simulink model "StraightWithLeadingCar_cs"  (R2016a)
settings: Solver=ode5  SolverMode=SingleTasking  StartTime=0.0  StopTime=40  FixedStep=1/1000  RelTol=1e-3
PreLoadFcn:
  | mbxruntime.callbacks.PreLoadFcn(bdroot);
PostLoadFcn:
  | mbxruntime.callbacks.PostLoadFcn(bdroot);
InitFcn:
  | mbxruntime.callbacks.InitFcn(bdroot);
StartFcn:
  | mbxruntime.callbacks.StartFcn(bdroot);
StopFcn:
  | mbxruntime.callbacks.StopFcn(bdroot);
model workspace (MAT data in the model file):
  mbox_table : struct (value not decoded)
  model_closed = 0
  sim_status = 0
values from neighbouring files (symbols this model uses):
  ACCDuration = 5    [PreScan_Runscript.m]
  V0 = ACCArray(2*ACCCasei-1)    [PreScan_Runscript.m]
  V1 = ACCArray(2*ACCCasei)    [PreScan_Runscript.m]
  VAccuracyIn = 0.8    [PreScan_Runscript.m]
  VDurationIn = 2    [PreScan_Runscript.m]
  VPIDIn = ACCArray(2*ACCCasei-1)    [PreScan_Runscript.m]
  VToleranceIn = 1    [PreScan_Runscript.m]
undefined symbols (not defined in the file or in its folder): ADASID, BMotor1, BMotor2, BrkDelayTime, DControlB, Delay1, Delay2, DiscIntNeverNeededParam, IControlB, JMotor1, JMotor2, mbxruntime, PControlB, PreScanCarSimLoadFcn, ratioGearF, ratioGearR, tabledata, TorqDelayTime, Tstep
undefined symbols (not defined in the file): SteeringColumn, SteeringWheel, WheelL0, WheelL1, WheelR0, WheelR1
libraries: simulink x14, simulink_extras x11, PreScanSimulinkLibrary x9, MyLib x3, Solver_SF x2, PreScanUsefulBlocks x2, pil_lib x1
(part 10 of 12)

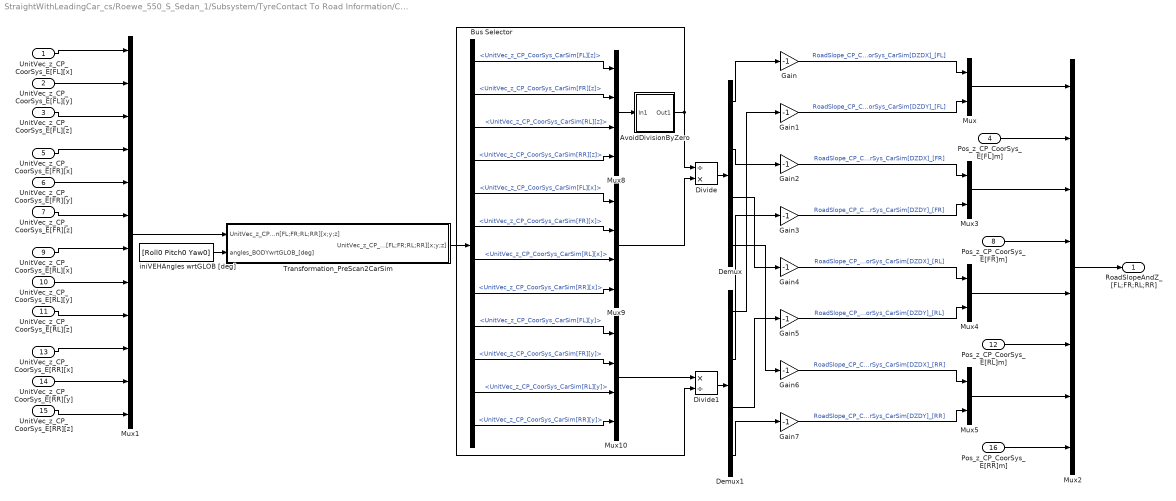
== system StraightWithLeadingCar_cs/Roewe_550_S_Sedan_1/Subsystem/TyreContact To Road Information/Contact To Road Information ==
  UnitVec_z_CP_CoorSys_E[FL][x] : Inport
  UnitVec_z_CP_CoorSys_E[FL][y] : Inport  Port=2
  UnitVec_z_CP_CoorSys_E[FL][z] : Inport  Port=3
  " Pos_z_CP_CoorSys_E[FL]m]" : Inport  Port=4
  UnitVec_z_CP_CoorSys_E[FR][x] : Inport  Port=5
  UnitVec_z_CP_CoorSys_E[FR][y] : Inport  Port=6
  UnitVec_z_CP_CoorSys_E[FR][z] : Inport  Port=7
  " Pos_z_CP_CoorSys_E[FR]m]" : Inport  Port=8
  UnitVec_z_CP_CoorSys_E[RL][x] : Inport  Port=9
  UnitVec_z_CP_CoorSys_E[RL][y] : Inport  Port=10
  UnitVec_z_CP_CoorSys_E[RL][z] : Inport  Port=11
  " Pos_z_CP_CoorSys_E[RL]m]" : Inport  Port=12
  UnitVec_z_CP_CoorSys_E[RR][x] : Inport  Port=13
  UnitVec_z_CP_CoorSys_E[RR][y] : Inport  Port=14
  UnitVec_z_CP_CoorSys_E[RR][z] : Inport  Port=15
  " Pos_z_CP_CoorSys_E[RR]m]" : Inport  Port=16
  AvoidDivisionByZero : Subsystem
  Bus Selector : BusSelector  OutputSignals=UnitVec_z_CP_CoorSys_CarSim[FL][x;y;z].UnitVec_z_CP_CoorSys_CarSim[FL][z],UnitVec_z_CP_CoorSys_CarSim[FR][x;y;z].UnitVec_z_CP_CoorSys_CarSim[FR][z],UnitVec_z_CP_CoorSys_CarSim[RL][x;y;z].UnitVec_z_CP_CoorSys_CarSim[RL][z],UnitVec_z_CP_CoorSys_CarSim[RR][x;y;z].UnitVec_z_CP_CoorSys_CarSim[RR][z],UnitVec_z_CP_CoorSys_CarSim[FL][x;y;z].UnitVec_z_CP_CoorSys_CarSim[FL][x],UnitVec_z_CP_CoorSys_CarSim[FR][x;y;z].UnitVec_z_CP_CoorSys_CarSim[FR][x],UnitVec_z_CP_CoorSys_CarSim[RL][x;y;z].UnitVec_z_CP_CoorSys_CarSim[RL][x],UnitVec_z_CP_CoorSys_CarSim[RR][x;y;z].UnitVec_z_CP_CoorSys_CarSim[RR][x],UnitVec_z_CP_CoorSys_CarSim[FL][x;y;z].UnitVec_z_CP_CoorSys_CarSim[FL][y],UnitVec_z_CP_CoorSys_CarSim[FR][x;y;z].UnitVec_z_CP_CoorSys_CarSim[FR][y],UnitVec_z_CP_CoorSys_CarSim[RL][x;y;z].UnitVec_z_CP_CoorSys_CarSim[RL][y],UnitVec_z_CP_CoorSys_CarSim[RR][x;y;z].UnitVec_z_CP_CoorSys_CarSim[RR][y]
  Demux : Demux
  Demux1 : Demux
  Divide : Product  Inputs=/*
  Divide1 : Product  Inputs=*/
  Gain{,1..7} (8 alike) : Gain  Gain=-1
  Mux{,3..5} (4 alike) : Mux  Inputs=2
  Mux1 : Mux  Inputs=12
  Mux10 : Mux
  Mux2 : Mux  Inputs=[2 1 2 1 2 1 2 1]
  Mux8 : Mux
  Mux9 : Mux
  Transformation_PreScan2CarSim : Subsystem
  iniVEHAngles wrtGLOB [deg] : Constant  Value=[Roll0 Pitch0 Yaw0]
  RoadSlopeAndZ_[FL;FR;RL;RR] : Outport
  wires:
  AvoidDivisionByZero/1(Out1) -> Divide1/2, Divide/1
  Demux1/4 -> Gain7/1
  Demux/4 -> Gain6/1
  Demux1/3 -> Gain5/1
  Demux/3 -> Gain4/1
  Demux1/2 -> Gain3/1
  Demux/2 -> Gain2/1
  Demux/1 -> Gain/1
  Demux1/1 -> Gain1/1
  Divide1/1 -> Demux1/1
  Divide/1 -> Demux/1
  Mux10/1 -> Divide1/1
  Mux9/1 -> Divide/2
  Mux8/1 -> AvoidDivisionByZero/1(In1)
  Bus Selector/12 -> Mux10/4  "<UnitVec_z_CP_CoorSys_CarSim[RR][y]>"
  Bus Selector/11 -> Mux10/3  "<UnitVec_z_CP_CoorSys_CarSim[RL][y]>"
  Bus Selector/10 -> Mux10/2  "<UnitVec_z_CP_CoorSys_CarSim[FR][y]>"
  Bus Selector/9 -> Mux10/1  "<UnitVec_z_CP_CoorSys_CarSim[FL][y]>"
  Bus Selector/8 -> Mux9/4  "<UnitVec_z_CP_CoorSys_CarSim[RR][x]>"
  Bus Selector/7 -> Mux9/3  "<UnitVec_z_CP_CoorSys_CarSim[RL][x]>"
  Bus Selector/6 -> Mux9/2  "<UnitVec_z_CP_CoorSys_CarSim[FR][x]>"
  Bus Selector/5 -> Mux9/1  "<UnitVec_z_CP_CoorSys_CarSim[FL][x]>"
  Bus Selector/4 -> Mux8/4  "<UnitVec_z_CP_CoorSys_CarSim[RR][z]>"
  Bus Selector/3 -> Mux8/3  "<UnitVec_z_CP_CoorSys_CarSim[RL][z]>"
  Bus Selector/2 -> Mux8/2  "<UnitVec_z_CP_CoorSys_CarSim[FR][z]>"
  Bus Selector/1 -> Mux8/1  "<UnitVec_z_CP_CoorSys_CarSim[FL][z]>"
  Mux5/1 -> Mux2/7
  Mux4/1 -> Mux2/5
  Mux3/1 -> Mux2/3
  " Pos_z_CP_CoorSys_E[FL]m]"/1 -> Mux2/2
  Mux/1 -> Mux2/1
  Gain/1 -> Mux/1  "RoadSlope_CP_CoorSys_CarSim[DZDX]_[FL]"
  " Pos_z_CP_CoorSys_E[RR]m]"/1 -> Mux2/8
  " Pos_z_CP_CoorSys_E[RL]m]"/1 -> Mux2/6
  " Pos_z_CP_CoorSys_E[FR]m]"/1 -> Mux2/4
  Transformation_PreScan2CarSim/1(UnitVec_z_CP_CoorSys _CarSim[FL;FR;RL;RR][x;y;z]) -> Bus Selector/1
  UnitVec_z_CP_CoorSys_E[RR][z]/1 -> Mux1/12
  UnitVec_z_CP_CoorSys_E[RR][y]/1 -> Mux1/11
  UnitVec_z_CP_CoorSys_E[RR][x]/1 -> Mux1/10
  UnitVec_z_CP_CoorSys_E[RL][z]/1 -> Mux1/9
  UnitVec_z_CP_CoorSys_E[RL][y]/1 -> Mux1/8
  UnitVec_z_CP_CoorSys_E[RL][x]/1 -> Mux1/7
  UnitVec_z_CP_CoorSys_E[FR][z]/1 -> Mux1/6
  UnitVec_z_CP_CoorSys_E[FR][y]/1 -> Mux1/5
  UnitVec_z_CP_CoorSys_E[FR][x]/1 -> Mux1/4
  UnitVec_z_CP_CoorSys_E[FL][z]/1 -> Mux1/3
  UnitVec_z_CP_CoorSys_E[FL][y]/1 -> Mux1/2
  UnitVec_z_CP_CoorSys_E[FL][x]/1 -> Mux1/1
  Mux1/1 -> Transformation_PreScan2CarSim/1(UnitVec_z_CP_CoorSys_PreScan[FL;FR;RL;RR][x;y;z])
  iniVEHAngles wrtGLOB [deg]/1 -> Transformation_PreScan2CarSim/2(angles_BODYwrtGLOB_[deg])
  Mux2/1 -> RoadSlopeAndZ_[FL;FR;RL;RR]/1
  Gain1/1 -> Mux/2  "RoadSlope_CP_CoorSys_CarSim[DZDY]_[FL]"
  Gain2/1 -> Mux3/1  "RoadSlope_CP_CoorSys_CarSim[DZDX]_[FR]"
  Gain3/1 -> Mux3/2  "RoadSlope_CP_CoorSys_CarSim[DZDY]_[FR]"
  Gain4/1 -> Mux4/1  "RoadSlope_CP_CoorSys_CarSim[DZDX]_[RL]"
  Gain5/1 -> Mux4/2  "RoadSlope_CP_CoorSys_CarSim[DZDY]_[RL]"
  Gain6/1 -> Mux5/1  "RoadSlope_CP_CoorSys_CarSim[DZDX]_[RR]"
  Gain7/1 -> Mux5/2  "RoadSlope_CP_CoorSys_CarSim[DZDY]_[RR]"

== system StraightWithLeadingCar_cs/Roewe_550_S_Sedan_1/Subsystem1/CarSim2PreScanSTATE/Transformation_SprungMassCarSim2PreScan ==
  In1 : Inport
  Demux : Demux  Outputs=3
  Ini z-position VEHICLE wrt GLOBAL axis system [m] : Constant  Value=z0
  Mux : Mux  Inputs=3
  Sum1 : Sum  Inputs=+-
  Out1 : Outport
  wires:
  Mux/1 -> Out1/1
  Ini z-position VEHICLE wrt GLOBAL axis system [m]/1 -> Sum1/2
  Demux/1 -> Mux/1
  Sum1/1 -> Mux/3
  Demux/3 -> Sum1/1
  Demux/2 -> Mux/2
  In1/1 -> Demux/1

== system StraightWithLeadingCar_cs/Roewe_550_S_Sedan_1/Subsystem1/CarSim2PreScan_BUS/Steering ==
  SteeringWheel_In : Inport
  AvoidDivisionByZero : Subsystem
  Bus Creator4 : BusCreator  Inputs=1
  DefaultValue : Constant  Value=16
  Demux2 : Demux  Outputs=2
  Divide : Product  Inputs=*/
  Switch : Switch  Criteria=u2 ~= 0
  Steering : Outport
  wires:
  AvoidDivisionByZero/1(Out1) -> Divide/2
  Switch/1 -> Bus Creator4/1  "SteeringRatio_[-]"
  DefaultValue/1 -> Switch/3
  Divide/1 -> Switch/1, Switch/2  "Steering_Ration[-]"
  Demux2/2 -> AvoidDivisionByZero/1(In1)  "Axle1ReducedSW"
  Demux2/1 -> Divide/1  "SteeringWheelAngle_[deg]"
  Bus Creator4/1 -> Steering/1  "Steering"
  SteeringWheel_In/1 -> Demux2/1

== system StraightWithLeadingCar_cs/Roewe_550_S_Sedan_1/Subsystem1/CarSim2PreScan_BUS/Vehicle ==
  v_VehicleCoG[x;y;z][km|h] : Inport
  Bus Creator1 : BusCreator  Inputs=1
  Bus Creator7 : BusCreator  Inputs=1
  Bus Creator8 : BusCreator  Inputs=3
  Demux : Demux  Outputs=3
  Vehicle : Outport
  wires:
  Demux/3 -> Bus Creator8/3  "v_Vehicle[z][km|h]"
  Demux/2 -> Bus Creator8/2  "v_Vehicle[y][km|h]"
  Demux/1 -> Bus Creator8/1  "v_Vehicle[x][km|h]"
  Bus Creator7/1 -> Bus Creator1/1  "Velocities"
  Bus Creator8/1 -> Bus Creator7/1  "Linear"
  Bus Creator1/1 -> Vehicle/1  "Vehicle"
  v_VehicleCoG[x;y;z][km|h]/1 -> Demux/1

== system StraightWithLeadingCar_cs/Roewe_550_S_Sedan_1/Subsystem1/CarSim2PreScan_BUS/Wheel ==
  SprungMass_Pos_Global[x;y;z][m] : Inport
  SprungMass_Angle_Global[x;y;z][deg] : Inport  Port=2
  CarSim_Pos_Wheel_[FL;FR;RL;RR][x;y;z][m] : Inport  Port=3
  CarSim_Angle_Wheel_[FL;FR;RL;RR][x;y;z][deg;rev;deg] : Inport  Port=4
  Bus Creator3 : BusCreator  Inputs=2
  Bus Creator6 : BusCreator  Inputs=1
  Convert CarSim to PreScan Wheel Position : Subsystem
  Convert CarSim to PreScan Wheel Rotation : Subsystem
  Demux : Demux  Outputs=[3 3 3 3]
  Demux1 : Demux  Outputs=[3 3 3 3]
  Wheel : Outport
  wires:
  SprungMass_Angle_Global[x;y;z][deg]/1 -> Convert CarSim to PreScan Wheel Rotation/5(Angle_Vehicle[x;y;z][deg]), Convert CarSim to PreScan Wheel Position/2(SprungMass_Angle_Global[x;y;z][deg])
  SprungMass_Pos_Global[x;y;z][m]/1 -> Convert CarSim to PreScan Wheel Position/1(SprungMass_Pos_Global[x;y;z][m])
  CarSim_Angle_Wheel_[FL;FR;RL;RR][x;y;z][deg;rev;deg]/1 -> Demux1/1
  Demux1/4 -> Convert CarSim to PreScan Wheel Rotation/4(CarSim_Angle_RR_Wheel_CoorSys_V[deg;rev;deg])  "CarSim_Angle_RR_Wheel_CoorSys_V[deg;rev;deg]"
  Demux1/3 -> Convert CarSim to PreScan Wheel Rotation/3(CarSim_Angle_RL_Wheel_CoorSys_V[deg;rev;deg])  "CarSim_Angle_RL_Wheel_CoorSys_V[deg;rev;deg]"
  Demux1/2 -> Convert CarSim to PreScan Wheel Rotation/2(CarSim_Angle_FR_Wheel_CoorSys_V[deg;rev;deg])  "CarSim_Angle_FR_Wheel_CoorSys_V[deg;rev;deg]"
  Demux1/1 -> Convert CarSim to PreScan Wheel Rotation/1(CarSim_Angle_FL_Wheel_CoorSys_V[deg;rev;deg])  "CarSim_Angle_FL_Wheel_CoorSys_V[deg;rev;deg]"
  CarSim_Pos_Wheel_[FL;FR;RL;RR][x;y;z][m]/1 -> Demux/1
  Demux/4 -> Convert CarSim to PreScan Wheel Position/6(CarSim_Pos_RR_Wheel[x;y;z][m])  "CarSim_Pos_RR_Wheel[x;y;z][m]"
  Demux/3 -> Convert CarSim to PreScan Wheel Position/5(CarSim_Pos_RL_Wheel[x;y;z][m])  "CarSim_Pos_RL_Wheel[x;y;z][m]"
  Demux/2 -> Convert CarSim to PreScan Wheel Position/4(CarSim_Pos_FR_Wheel[x;y;z][m])  "CarSim_Pos_FR_Wheel[x;y;z][m]"
  Demux/1 -> Convert CarSim to PreScan Wheel Position/3(CarSim_Pos_FL_Wheel[x;y;z][m])  "CarSim_Pos_FL_Wheel[x;y;z][m]"
  Bus Creator6/1 -> Wheel/1  "Wheel"
  Bus Creator3/1 -> Bus Creator6/1  "Position"
  Convert CarSim to PreScan Wheel Rotation/1(PreScanWheel_Rot) -> Bus Creator3/2
  Convert CarSim to PreScan Wheel Position/1(PreScanWheel_Pos) -> Bus Creator3/1

== system StraightWithLeadingCar_cs/BMW_X5_SUV_1/Trajectories/Traj2State1/Traj2State2/MuxState ==
  x [m] : Inport
  y [m] : Inport  Port=2
  z [m] : Inport  Port=3
  dx [m/s] : Inport  Port=4
  dy [m/s] : Inport  Port=5
  dz [m/s] : Inport  Port=6
  R [rad] : Inport  Port=7
  P [rad] : Inport  Port=8
  Y [rad] : Inport  Port=9
  Mux : Mux  Inputs=9
  state : Outport
  wires:
  z [m]/1 -> Mux/3
  y [m]/1 -> Mux/2
  x [m]/1 -> Mux/1
  Y [rad]/1 -> Mux/9
  P [rad]/1 -> Mux/8
  R [rad]/1 -> Mux/7
  dz [m/s]/1 -> Mux/6
  dy [m/s]/1 -> Mux/5
  dx [m/s]/1 -> Mux/4
  Mux/1 -> state/1

== system StraightWithLeadingCar_cs/BMW_X5_SUV_1/Trajectories/Traj2State1/Traj2State2/Traj2MuxState_Ext ==
  Traj : Inport
  Terminator{1..9} (9 alike) : Terminator
  demux : Subsystem
  x [m] : Outport
  y [m] : Outport  Port=2
  z [m] : Outport  Port=3
  dx [m/s] : Outport  Port=4
  dy [m/s] : Outport  Port=5
  dz [m/s] : Outport  Port=6
  R [rad] : Outport  Port=7
  P [rad] : Outport  Port=8
  Y [rad] : Outport  Port=9
  wires:
  demux/9(Y) -> Y [rad]/1
  demux/7(R) -> R [rad]/1
  demux/5(vely) -> dy [m/s]/1
  demux/4(velx) -> dx [m/s]/1
  demux/10(velR) -> Terminator4/1
  demux/11(velP) -> Terminator5/1
  demux/12(velY) -> Terminator1/1
  demux/13(accx) -> Terminator8/1
  demux/14(accy) -> Terminator9/1
  demux/15(accz) -> Terminator7/1
  demux/18(accY) -> Terminator2/1
  demux/16(accR) -> Terminator3/1
  demux/17(accP) -> Terminator6/1
  demux/3(z) -> z [m]/1
  Traj/1 -> demux/1(traj)
  demux/6(velz) -> dz [m/s]/1
  demux/1(x) -> x [m]/1
  demux/2(y) -> y [m]/1
  demux/8(P) -> P [rad]/1

== system StraightWithLeadingCar_cs/Roewe_550_S_Sedan_1/CarSim I//O/PreScanLaneMarker/Subsystem/Sensor Data ==
  Sensor Data : Inport
  Bus Selector : BusSelector  OutputSignals=ScanAtSensor.LeftLaneIntersection2.WorldCoordinateY,ScanAtDistance1.LeftLaneIntersection2.WorldCoordinateY,ScanAtDistance2.LeftLaneIntersection2.WorldCoordinateY,ScanAtDistance3.LeftLaneIntersection2.WorldCoordinateY
  Bus Selector1 : BusSelector  OutputSignals=ScanAtSensor.LeftLaneIntersection1.WorldCoordinateY,ScanAtDistance1.LeftLaneIntersection1.WorldCoordinateY,ScanAtDistance2.LeftLaneIntersection1.WorldCoordinateY,ScanAtDistance3.LeftLaneIntersection1.WorldCoordinateY
  Bus Selector2 : BusSelector  OutputSignals=ScanAtSensor.RightLaneIntersection1.WorldCoordinateY,ScanAtDistance1.RightLaneIntersection1.WorldCoordinateY,ScanAtDistance2.RightLaneIntersection1.WorldCoordinateY,ScanAtDistance3.RightLaneIntersection1.WorldCoordinateY
  Bus Selector3 : BusSelector  OutputSignals=ScanAtSensor.RightLaneIntersection2.WorldCoordinateX,ScanAtDistance1.RightLaneIntersection2.WorldCoordinateX,ScanAtDistance2.RightLaneIntersection2.WorldCoordinateX,ScanAtDistance3.RightLaneIntersection2.WorldCoordinateX
  Bus Selector4 : BusSelector  OutputSignals=ScanAtSensor.SliceCenterCoordsX,ScanAtSensor.SliceCenterCoordsY
  Bus Selector5 : BusSelector  OutputSignals=ScanAtSensor.LeftLaneIntersection2.WorldCoordinateX,ScanAtDistance1.LeftLaneIntersection2.WorldCoordinateX,ScanAtDistance2.LeftLaneIntersection2.WorldCoordinateX,ScanAtDistance3.LeftLaneIntersection2.WorldCoordinateX
  Bus Selector6 : BusSelector  OutputSignals=ScanAtSensor.LeftLaneIntersection1.WorldCoordinateX,ScanAtDistance1.LeftLaneIntersection1.WorldCoordinateX,ScanAtDistance2.LeftLaneIntersection1.WorldCoordinateX,ScanAtDistance3.LeftLaneIntersection1.WorldCoordinateX
  Bus Selector7 : BusSelector  OutputSignals=ScanAtSensor.RightLaneIntersection1.WorldCoordinateX,ScanAtDistance1.RightLaneIntersection1.WorldCoordinateX,ScanAtDistance2.RightLaneIntersection1.WorldCoordinateX,ScanAtDistance3.RightLaneIntersection1.WorldCoordinateX
  Bus Selector8 : BusSelector  OutputSignals=ScanAtSensor.RightLaneIntersection2.WorldCoordinateY,ScanAtDistance1.RightLaneIntersection2.WorldCoordinateY,ScanAtDistance2.RightLaneIntersection2.WorldCoordinateY,ScanAtDistance3.RightLaneIntersection2.WorldCoordinateY
  Mux{,1..7} (8 alike) : Mux
  X0 : Outport
  Y0 : Outport  Port=2
  Lane3_X_Part0 : Outport  Port=3
  Lane1_X_Part0 : Outport  Port=4
  Lane2_X_Part0 : Outport  Port=5
  Lane4_X_Part0 : Outport  Port=6
  Lane3_Y_Part0 : Outport  Port=7
  Lane1_Y_Part0 : Outport  Port=8
  Lane2_Y_Part0 : Outport  Port=9
  Lane4_Y_Part0 : Outport  Port=10
  wires:
  Sensor Data/1 -> Bus Selector8/1, Bus Selector2/1, Bus Selector1/1, Bus Selector/1, Bus Selector3/1, Bus Selector5/1, Bus Selector4/1, Bus Selector6/1, Bus Selector7/1
  Bus Selector4/2 -> Y0/1  "<SliceCenterCoordsY>"
  Bus Selector4/1 -> X0/1  "<SliceCenterCoordsX>"
  Bus Selector5/2 -> Mux/2  "<WorldCoordinateX>"
  Bus Selector5/4 -> Mux/4  "<WorldCoordinateX>"
  Bus Selector5/1 -> Mux/1  "<WorldCoordinateX>"
  Bus Selector5/3 -> Mux/3  "<WorldCoordinateX>"
  Bus Selector/3 -> Mux4/3  "<WorldCoordinateY>"
  Bus Selector/4 -> Mux4/4  "<WorldCoordinateY>"
  Bus Selector/1 -> Mux4/1  "<WorldCoordinateY>"
  Bus Selector/2 -> Mux4/2  "<WorldCoordinateY>"
  Mux/1 -> Lane3_X_Part0/1
  Mux4/1 -> Lane3_Y_Part0/1
  Bus Selector6/4 -> Mux5/4  "<WorldCoordinateX>"
  Bus Selector6/3 -> Mux5/3  "<WorldCoordinateX>"
  Bus Selector6/2 -> Mux5/2  "<WorldCoordinateX>"
  Bus Selector6/1 -> Mux5/1  "<WorldCoordinateX>"
  Bus Selector1/3 -> Mux1/3  "<WorldCoordinateY>"
  Bus Selector1/2 -> Mux1/2  "<WorldCoordinateY>"
  Bus Selector1/4 -> Mux1/4  "<WorldCoordinateY>"
  Bus Selector1/1 -> Mux1/1  "<WorldCoordinateY>"
  Mux1/1 -> Lane1_Y_Part0/1
  Mux5/1 -> Lane1_X_Part0/1
  Bus Selector7/2 -> Mux2/2  "<WorldCoordinateX>"
  Bus Selector7/3 -> Mux2/3  "<WorldCoordinateX>"
  Bus Selector7/1 -> Mux2/1  "<WorldCoordinateX>"
  Bus Selector7/4 -> Mux2/4  "<WorldCoordinateX>"
  Bus Selector2/2 -> Mux3/2  "<WorldCoordinateY>"
  Bus Selector2/1 -> Mux3/1  "<WorldCoordinateY>"
  Bus Selector2/3 -> Mux3/3  "<WorldCoordinateY>"
  Bus Selector2/4 -> Mux3/4  "<WorldCoordinateY>"
  Bus Selector3/2 -> Mux6/2  "<WorldCoordinateX>"
  Bus Selector3/1 -> Mux6/1  "<WorldCoordinateX>"
  Bus Selector3/3 -> Mux6/3  "<WorldCoordinateX>"
  Bus Selector3/4 -> Mux6/4  "<WorldCoordinateX>"
  Bus Selector8/1 -> Mux7/1  "<WorldCoordinateY>"
  Bus Selector8/2 -> Mux7/2  "<WorldCoordinateY>"
  Bus Selector8/3 -> Mux7/3  "<WorldCoordinateY>"
  Bus Selector8/4 -> Mux7/4  "<WorldCoordinateY>"
  Mux3/1 -> Lane2_Y_Part0/1
  Mux7/1 -> Lane4_Y_Part0/1
  Mux2/1 -> Lane2_X_Part0/1
  Mux6/1 -> Lane4_X_Part0/1

== system StraightWithLeadingCar_cs/Roewe_550_S_Sedan_1/CarSim I//O/PreScanLaneMarker/Subsystem/Sensor Data1 ==
  Sensor Data : Inport
  Bus Selector : BusSelector  OutputSignals=ScanAtSensor.LeftLaneIntersection2.WorldCoordinateY,ScanAtDistance1.LeftLaneIntersection2.WorldCoordinateY,ScanAtDistance2.LeftLaneIntersection2.WorldCoordinateY,ScanAtDistance3.LeftLaneIntersection2.WorldCoordinateY
  Bus Selector1 : BusSelector  OutputSignals=ScanAtSensor.LeftLaneIntersection1.WorldCoordinateY,ScanAtDistance1.LeftLaneIntersection1.WorldCoordinateY,ScanAtDistance2.LeftLaneIntersection1.WorldCoordinateY,ScanAtDistance3.LeftLaneIntersection1.WorldCoordinateY
  Bus Selector2 : BusSelector  OutputSignals=ScanAtSensor.RightLaneIntersection1.WorldCoordinateY,ScanAtDistance1.RightLaneIntersection1.WorldCoordinateY,ScanAtDistance2.RightLaneIntersection1.WorldCoordinateY,ScanAtDistance3.RightLaneIntersection1.WorldCoordinateY
  Bus Selector3 : BusSelector  OutputSignals=ScanAtSensor.RightLaneIntersection2.WorldCoordinateX,ScanAtDistance1.RightLaneIntersection2.WorldCoordinateX,ScanAtDistance2.RightLaneIntersection2.WorldCoordinateX,ScanAtDistance3.RightLaneIntersection2.WorldCoordinateX
  Bus Selector5 : BusSelector  OutputSignals=ScanAtSensor.LeftLaneIntersection2.WorldCoordinateX,ScanAtDistance1.LeftLaneIntersection2.WorldCoordinateX,ScanAtDistance2.LeftLaneIntersection2.WorldCoordinateX,ScanAtDistance3.LeftLaneIntersection2.WorldCoordinateX
  Bus Selector6 : BusSelector  OutputSignals=ScanAtSensor.LeftLaneIntersection1.WorldCoordinateX,ScanAtDistance1.LeftLaneIntersection1.WorldCoordinateX,ScanAtDistance2.LeftLaneIntersection1.WorldCoordinateX,ScanAtDistance3.LeftLaneIntersection1.WorldCoordinateX
  Bus Selector7 : BusSelector  OutputSignals=ScanAtSensor.RightLaneIntersection1.WorldCoordinateX,ScanAtDistance1.RightLaneIntersection1.WorldCoordinateX,ScanAtDistance2.RightLaneIntersection1.WorldCoordinateX,ScanAtDistance3.RightLaneIntersection1.WorldCoordinateX
  Bus Selector8 : BusSelector  OutputSignals=ScanAtSensor.RightLaneIntersection2.WorldCoordinateY,ScanAtDistance1.RightLaneIntersection2.WorldCoordinateY,ScanAtDistance2.RightLaneIntersection2.WorldCoordinateY,ScanAtDistance3.RightLaneIntersection2.WorldCoordinateY
  Mux{,1..7} (8 alike) : Mux
  Lane3_X_Part1 : Outport
  Lane1_X_Part1 : Outport  Port=2
  Lane2_X_Part1 : Outport  Port=3
  Lane4_X_Part1 : Outport  Port=4
  Lane3_Y_Part1 : Outport  Port=5
  Lane1_Y_Part1 : Outport  Port=6
  Lane2_Y_Part1 : Outport  Port=7
  Lane4_Y_Part1 : Outport  Port=8
  wires:
  Sensor Data/1 -> Bus Selector8/1, Bus Selector2/1, Bus Selector1/1, Bus Selector/1, Bus Selector3/1, Bus Selector5/1, Bus Selector6/1, Bus Selector7/1
  Bus Selector5/2 -> Mux/2  "<WorldCoordinateX>"
  Bus Selector5/4 -> Mux/4  "<WorldCoordinateX>"
  Bus Selector5/1 -> Mux/1  "<WorldCoordinateX>"
  Bus Selector5/3 -> Mux/3  "<WorldCoordinateX>"
  Bus Selector/3 -> Mux4/3  "<WorldCoordinateY>"
  Bus Selector/4 -> Mux4/4  "<WorldCoordinateY>"
  Bus Selector/1 -> Mux4/1  "<WorldCoordinateY>"
  Bus Selector/2 -> Mux4/2  "<WorldCoordinateY>"
  Mux/1 -> Lane3_X_Part1/1
  Mux4/1 -> Lane3_Y_Part1/1
  Bus Selector6/4 -> Mux5/4  "<WorldCoordinateX>"
  Bus Selector6/3 -> Mux5/3  "<WorldCoordinateX>"
  Bus Selector6/2 -> Mux5/2  "<WorldCoordinateX>"
  Bus Selector6/1 -> Mux5/1  "<WorldCoordinateX>"
  Bus Selector1/3 -> Mux1/3  "<WorldCoordinateY>"
  Bus Selector1/2 -> Mux1/2  "<WorldCoordinateY>"
  Bus Selector1/4 -> Mux1/4  "<WorldCoordinateY>"
  Bus Selector1/1 -> Mux1/1  "<WorldCoordinateY>"
  Mux1/1 -> Lane1_Y_Part1/1
  Mux5/1 -> Lane1_X_Part1/1
  Bus Selector7/2 -> Mux2/2  "<WorldCoordinateX>"
  Bus Selector7/3 -> Mux2/3  "<WorldCoordinateX>"
  Bus Selector7/1 -> Mux2/1  "<WorldCoordinateX>"
  Bus Selector7/4 -> Mux2/4  "<WorldCoordinateX>"
  Bus Selector2/2 -> Mux3/2  "<WorldCoordinateY>"
  Bus Selector2/1 -> Mux3/1  "<WorldCoordinateY>"
  Bus Selector2/3 -> Mux3/3  "<WorldCoordinateY>"
  Bus Selector2/4 -> Mux3/4  "<WorldCoordinateY>"
  Bus Selector3/2 -> Mux6/2  "<WorldCoordinateX>"
  Bus Selector3/1 -> Mux6/1  "<WorldCoordinateX>"
  Bus Selector3/3 -> Mux6/3  "<WorldCoordinateX>"
  Bus Selector3/4 -> Mux6/4  "<WorldCoordinateX>"
  Bus Selector8/1 -> Mux7/1  "<WorldCoordinateY>"
  Bus Selector8/2 -> Mux7/2  "<WorldCoordinateY>"
  Bus Selector8/3 -> Mux7/3  "<WorldCoordinateY>"
  Bus Selector8/4 -> Mux7/4  "<WorldCoordinateY>"
  Mux3/1 -> Lane2_Y_Part1/1
  Mux7/1 -> Lane4_Y_Part1/1
  Mux2/1 -> Lane2_X_Part1/1
  Mux6/1 -> Lane4_X_Part1/1

== system StraightWithLeadingCar_cs/Roewe_550_S_Sedan_1/CarSim I//O/PreScanLaneMarker/Subsystem/Sensor Data2 ==
  Sensor Data : Inport
  Bus Selector : BusSelector  OutputSignals=ScanAtSensor.LeftLaneIntersection2.WorldCoordinateY,ScanAtDistance1.LeftLaneIntersection2.WorldCoordinateY,ScanAtDistance2.LeftLaneIntersection2.WorldCoordinateY,ScanAtDistance3.LeftLaneIntersection2.WorldCoordinateY
  Bus Selector1 : BusSelector  OutputSignals=ScanAtSensor.LeftLaneIntersection1.WorldCoordinateY,ScanAtDistance1.LeftLaneIntersection1.WorldCoordinateY,ScanAtDistance2.LeftLaneIntersection1.WorldCoordinateY,ScanAtDistance3.LeftLaneIntersection1.WorldCoordinateY
  Bus Selector2 : BusSelector  OutputSignals=ScanAtSensor.RightLaneIntersection1.WorldCoordinateY,ScanAtDistance1.RightLaneIntersection1.WorldCoordinateY,ScanAtDistance2.RightLaneIntersection1.WorldCoordinateY,ScanAtDistance3.RightLaneIntersection1.WorldCoordinateY
  Bus Selector3 : BusSelector  OutputSignals=ScanAtSensor.RightLaneIntersection2.WorldCoordinateX,ScanAtDistance1.RightLaneIntersection2.WorldCoordinateX,ScanAtDistance2.RightLaneIntersection2.WorldCoordinateX,ScanAtDistance3.RightLaneIntersection2.WorldCoordinateX
  Bus Selector5 : BusSelector  OutputSignals=ScanAtSensor.LeftLaneIntersection2.WorldCoordinateX,ScanAtDistance1.LeftLaneIntersection2.WorldCoordinateX,ScanAtDistance2.LeftLaneIntersection2.WorldCoordinateX,ScanAtDistance3.LeftLaneIntersection2.WorldCoordinateX
  Bus Selector6 : BusSelector  OutputSignals=ScanAtSensor.LeftLaneIntersection1.WorldCoordinateX,ScanAtDistance1.LeftLaneIntersection1.WorldCoordinateX,ScanAtDistance2.LeftLaneIntersection1.WorldCoordinateX,ScanAtDistance3.LeftLaneIntersection1.WorldCoordinateX
  Bus Selector7 : BusSelector  OutputSignals=ScanAtSensor.RightLaneIntersection1.WorldCoordinateX,ScanAtDistance1.RightLaneIntersection1.WorldCoordinateX,ScanAtDistance2.RightLaneIntersection1.WorldCoordinateX,ScanAtDistance3.RightLaneIntersection1.WorldCoordinateX
  Bus Selector8 : BusSelector  OutputSignals=ScanAtSensor.RightLaneIntersection2.WorldCoordinateY,ScanAtDistance1.RightLaneIntersection2.WorldCoordinateY,ScanAtDistance2.RightLaneIntersection2.WorldCoordinateY,ScanAtDistance3.RightLaneIntersection2.WorldCoordinateY
  Mux{,1..7} (8 alike) : Mux
  Lane3_X_Part2 : Outport
  Lane1_X_Part2 : Outport  Port=2
  Lane2_X_Part2 : Outport  Port=3
  Lane4_X_Part2 : Outport  Port=4
  Lane3_Y_Part2 : Outport  Port=5
  Lane1_Y_Part2 : Outport  Port=6
  Lane2_Y_Part2 : Outport  Port=7
  Lane4_Y_Part2 : Outport  Port=8
  wires:
  Sensor Data/1 -> Bus Selector8/1, Bus Selector2/1, Bus Selector1/1, Bus Selector/1, Bus Selector3/1, Bus Selector5/1, Bus Selector6/1, Bus Selector7/1
  Bus Selector5/2 -> Mux/2  "<WorldCoordinateX>"
  Bus Selector5/4 -> Mux/4  "<WorldCoordinateX>"
  Bus Selector5/1 -> Mux/1  "<WorldCoordinateX>"
  Bus Selector5/3 -> Mux/3  "<WorldCoordinateX>"
  Bus Selector/3 -> Mux4/3  "<WorldCoordinateY>"
  Bus Selector/4 -> Mux4/4  "<WorldCoordinateY>"
  Bus Selector/1 -> Mux4/1  "<WorldCoordinateY>"
  Bus Selector/2 -> Mux4/2  "<WorldCoordinateY>"
  Mux/1 -> Lane3_X_Part2/1
  Mux4/1 -> Lane3_Y_Part2/1
  Bus Selector6/4 -> Mux5/4  "<WorldCoordinateX>"
  Bus Selector6/3 -> Mux5/3  "<WorldCoordinateX>"
  Bus Selector6/2 -> Mux5/2  "<WorldCoordinateX>"
  Bus Selector6/1 -> Mux5/1  "<WorldCoordinateX>"
  Bus Selector1/3 -> Mux1/3  "<WorldCoordinateY>"
  Bus Selector1/2 -> Mux1/2  "<WorldCoordinateY>"
  Bus Selector1/4 -> Mux1/4  "<WorldCoordinateY>"
  Bus Selector1/1 -> Mux1/1  "<WorldCoordinateY>"
  Mux1/1 -> Lane1_Y_Part2/1
  Mux5/1 -> Lane1_X_Part2/1
  Bus Selector7/2 -> Mux2/2  "<WorldCoordinateX>"
  Bus Selector7/3 -> Mux2/3  "<WorldCoordinateX>"
  Bus Selector7/1 -> Mux2/1  "<WorldCoordinateX>"
  Bus Selector7/4 -> Mux2/4  "<WorldCoordinateX>"
  Bus Selector2/2 -> Mux3/2  "<WorldCoordinateY>"
  Bus Selector2/1 -> Mux3/1  "<WorldCoordinateY>"
  Bus Selector2/3 -> Mux3/3  "<WorldCoordinateY>"
  Bus Selector2/4 -> Mux3/4  "<WorldCoordinateY>"
  Bus Selector3/2 -> Mux6/2  "<WorldCoordinateX>"
  Bus Selector3/1 -> Mux6/1  "<WorldCoordinateX>"
  Bus Selector3/3 -> Mux6/3  "<WorldCoordinateX>"
  Bus Selector3/4 -> Mux6/4  "<WorldCoordinateX>"
  Bus Selector8/1 -> Mux7/1  "<WorldCoordinateY>"
  Bus Selector8/2 -> Mux7/2  "<WorldCoordinateY>"
  Bus Selector8/3 -> Mux7/3  "<WorldCoordinateY>"
  Bus Selector8/4 -> Mux7/4  "<WorldCoordinateY>"
  Mux3/1 -> Lane2_Y_Part2/1
  Mux7/1 -> Lane4_Y_Part2/1
  Mux2/1 -> Lane2_X_Part2/1
  Mux6/1 -> Lane4_X_Part2/1

== system StraightWithLeadingCar_cs/Roewe_550_S_Sedan_1/CarSim I//O/PreScanLaneMarker/Subsystem/Sensor Data3 ==
  Sensor Data : Inport
  Bus Selector : BusSelector  OutputSignals=ScanAtSensor.LeftLaneIntersection2.WorldCoordinateY,ScanAtDistance1.LeftLaneIntersection2.WorldCoordinateY,ScanAtDistance2.LeftLaneIntersection2.WorldCoordinateY,ScanAtDistance3.LeftLaneIntersection2.WorldCoordinateY
  Bus Selector1 : BusSelector  OutputSignals=ScanAtSensor.LeftLaneIntersection1.WorldCoordinateY,ScanAtDistance1.LeftLaneIntersection1.WorldCoordinateY,ScanAtDistance2.LeftLaneIntersection1.WorldCoordinateY,ScanAtDistance3.LeftLaneIntersection1.WorldCoordinateY
  Bus Selector2 : BusSelector  OutputSignals=ScanAtSensor.RightLaneIntersection1.WorldCoordinateY,ScanAtDistance1.RightLaneIntersection1.WorldCoordinateY,ScanAtDistance2.RightLaneIntersection1.WorldCoordinateY,ScanAtDistance3.RightLaneIntersection1.WorldCoordinateY
  Bus Selector3 : BusSelector  OutputSignals=ScanAtSensor.RightLaneIntersection2.WorldCoordinateX,ScanAtDistance1.RightLaneIntersection2.WorldCoordinateX,ScanAtDistance2.RightLaneIntersection2.WorldCoordinateX,ScanAtDistance3.RightLaneIntersection2.WorldCoordinateX
  Bus Selector5 : BusSelector  OutputSignals=ScanAtSensor.LeftLaneIntersection2.WorldCoordinateX,ScanAtDistance1.LeftLaneIntersection2.WorldCoordinateX,ScanAtDistance2.LeftLaneIntersection2.WorldCoordinateX,ScanAtDistance3.LeftLaneIntersection2.WorldCoordinateX
  Bus Selector6 : BusSelector  OutputSignals=ScanAtSensor.LeftLaneIntersection1.WorldCoordinateX,ScanAtDistance1.LeftLaneIntersection1.WorldCoordinateX,ScanAtDistance2.LeftLaneIntersection1.WorldCoordinateX,ScanAtDistance3.LeftLaneIntersection1.WorldCoordinateX
  Bus Selector7 : BusSelector  OutputSignals=ScanAtSensor.RightLaneIntersection1.WorldCoordinateX,ScanAtDistance1.RightLaneIntersection1.WorldCoordinateX,ScanAtDistance2.RightLaneIntersection1.WorldCoordinateX,ScanAtDistance3.RightLaneIntersection1.WorldCoordinateX
  Bus Selector8 : BusSelector  OutputSignals=ScanAtSensor.RightLaneIntersection2.WorldCoordinateY,ScanAtDistance1.RightLaneIntersection2.WorldCoordinateY,ScanAtDistance2.RightLaneIntersection2.WorldCoordinateY,ScanAtDistance3.RightLaneIntersection2.WorldCoordinateY
  Mux{,1..7} (8 alike) : Mux
  Lane3_X_Part3 : Outport
  Lane1_X_Part3 : Outport  Port=2
  Lane2_X_Part3 : Outport  Port=3
  Lane4_X_Part3 : Outport  Port=4
  Lane3_Y_Part3 : Outport  Port=5
  Lane1_Y_Part3 : Outport  Port=6
  Lane2_Y_Part3 : Outport  Port=7
  Lane4_Y_Part3 : Outport  Port=8
  wires:
  Sensor Data/1 -> Bus Selector8/1, Bus Selector2/1, Bus Selector1/1, Bus Selector/1, Bus Selector3/1, Bus Selector5/1, Bus Selector6/1, Bus Selector7/1
  Bus Selector5/2 -> Mux/2  "<WorldCoordinateX>"
  Bus Selector5/4 -> Mux/4  "<WorldCoordinateX>"
  Bus Selector5/1 -> Mux/1  "<WorldCoordinateX>"
  Bus Selector5/3 -> Mux/3  "<WorldCoordinateX>"
  Bus Selector/3 -> Mux4/3  "<WorldCoordinateY>"
  Bus Selector/4 -> Mux4/4  "<WorldCoordinateY>"
  Bus Selector/1 -> Mux4/1  "<WorldCoordinateY>"
  Bus Selector/2 -> Mux4/2  "<WorldCoordinateY>"
  Mux/1 -> Lane3_X_Part3/1
  Mux4/1 -> Lane3_Y_Part3/1
  Bus Selector6/4 -> Mux5/4  "<WorldCoordinateX>"
  Bus Selector6/3 -> Mux5/3  "<WorldCoordinateX>"
  Bus Selector6/2 -> Mux5/2  "<WorldCoordinateX>"
  Bus Selector6/1 -> Mux5/1  "<WorldCoordinateX>"
  Bus Selector1/3 -> Mux1/3  "<WorldCoordinateY>"
  Bus Selector1/2 -> Mux1/2  "<WorldCoordinateY>"
  Bus Selector1/4 -> Mux1/4  "<WorldCoordinateY>"
  Bus Selector1/1 -> Mux1/1  "<WorldCoordinateY>"
  Mux1/1 -> Lane1_Y_Part3/1
  Mux5/1 -> Lane1_X_Part3/1
  Bus Selector7/2 -> Mux2/2  "<WorldCoordinateX>"
  Bus Selector7/3 -> Mux2/3  "<WorldCoordinateX>"
  Bus Selector7/1 -> Mux2/1  "<WorldCoordinateX>"
  Bus Selector7/4 -> Mux2/4  "<WorldCoordinateX>"
  Bus Selector2/2 -> Mux3/2  "<WorldCoordinateY>"
  Bus Selector2/1 -> Mux3/1  "<WorldCoordinateY>"
  Bus Selector2/3 -> Mux3/3  "<WorldCoordinateY>"
  Bus Selector2/4 -> Mux3/4  "<WorldCoordinateY>"
  Bus Selector3/2 -> Mux6/2  "<WorldCoordinateX>"
  Bus Selector3/1 -> Mux6/1  "<WorldCoordinateX>"
  Bus Selector3/3 -> Mux6/3  "<WorldCoordinateX>"
  Bus Selector3/4 -> Mux6/4  "<WorldCoordinateX>"
  Bus Selector8/1 -> Mux7/1  "<WorldCoordinateY>"
  Bus Selector8/2 -> Mux7/2  "<WorldCoordinateY>"
  Bus Selector8/3 -> Mux7/3  "<WorldCoordinateY>"
  Bus Selector8/4 -> Mux7/4  "<WorldCoordinateY>"
  Mux3/1 -> Lane2_Y_Part3/1
  Mux7/1 -> Lane4_Y_Part3/1
  Mux2/1 -> Lane2_X_Part3/1
  Mux6/1 -> Lane4_X_Part3/1

== system StraightWithLeadingCar_cs/Roewe_550_S_Sedan_1/CarSim I//O/PreScanLaneMarker/Subsystem/Sensor Data4 ==
  Sensor Data : Inport
  Bus Selector : BusSelector  OutputSignals=ScanAtSensor.LeftLaneIntersection2.WorldCoordinateY,ScanAtDistance1.LeftLaneIntersection2.WorldCoordinateY,ScanAtDistance2.LeftLaneIntersection2.WorldCoordinateY,ScanAtDistance3.LeftLaneIntersection2.WorldCoordinateY
  Bus Selector1 : BusSelector  OutputSignals=ScanAtSensor.LeftLaneIntersection1.WorldCoordinateY,ScanAtDistance1.LeftLaneIntersection1.WorldCoordinateY,ScanAtDistance2.LeftLaneIntersection1.WorldCoordinateY,ScanAtDistance3.LeftLaneIntersection1.WorldCoordinateY
  Bus Selector2 : BusSelector  OutputSignals=ScanAtSensor.RightLaneIntersection1.WorldCoordinateY,ScanAtDistance1.RightLaneIntersection1.WorldCoordinateY,ScanAtDistance2.RightLaneIntersection1.WorldCoordinateY,ScanAtDistance3.RightLaneIntersection1.WorldCoordinateY
  Bus Selector3 : BusSelector  OutputSignals=ScanAtSensor.RightLaneIntersection2.WorldCoordinateX,ScanAtDistance1.RightLaneIntersection2.WorldCoordinateX,ScanAtDistance2.RightLaneIntersection2.WorldCoordinateX,ScanAtDistance3.RightLaneIntersection2.WorldCoordinateX
  Bus Selector5 : BusSelector  OutputSignals=ScanAtSensor.LeftLaneIntersection2.WorldCoordinateX,ScanAtDistance1.LeftLaneIntersection2.WorldCoordinateX,ScanAtDistance2.LeftLaneIntersection2.WorldCoordinateX,ScanAtDistance3.LeftLaneIntersection2.WorldCoordinateX
  Bus Selector6 : BusSelector  OutputSignals=ScanAtSensor.LeftLaneIntersection1.WorldCoordinateX,ScanAtDistance1.LeftLaneIntersection1.WorldCoordinateX,ScanAtDistance2.LeftLaneIntersection1.WorldCoordinateX,ScanAtDistance3.LeftLaneIntersection1.WorldCoordinateX
  Bus Selector7 : BusSelector  OutputSignals=ScanAtSensor.RightLaneIntersection1.WorldCoordinateX,ScanAtDistance1.RightLaneIntersection1.WorldCoordinateX,ScanAtDistance2.RightLaneIntersection1.WorldCoordinateX,ScanAtDistance3.RightLaneIntersection1.WorldCoordinateX
  Bus Selector8 : BusSelector  OutputSignals=ScanAtSensor.RightLaneIntersection2.WorldCoordinateY,ScanAtDistance1.RightLaneIntersection2.WorldCoordinateY,ScanAtDistance2.RightLaneIntersection2.WorldCoordinateY,ScanAtDistance3.RightLaneIntersection2.WorldCoordinateY
  Mux{,1..7} (8 alike) : Mux
  Lane3_X_Part4 : Outport
  Lane1_X_Part4 : Outport  Port=2
  Lane2_X_Part4 : Outport  Port=3
  Lane4_X_Part4 : Outport  Port=4
  Lane3_Y_Part4 : Outport  Port=5
  Lane1_Y_Part4 : Outport  Port=6
  Lane2_Y_Part4 : Outport  Port=7
  Lane4_Y_Part4 : Outport  Port=8
  wires:
  Sensor Data/1 -> Bus Selector8/1, Bus Selector2/1, Bus Selector1/1, Bus Selector/1, Bus Selector3/1, Bus Selector5/1, Bus Selector6/1, Bus Selector7/1
  Bus Selector5/2 -> Mux/2  "<WorldCoordinateX>"
  Bus Selector5/4 -> Mux/4  "<WorldCoordinateX>"
  Bus Selector5/1 -> Mux/1  "<WorldCoordinateX>"
  Bus Selector5/3 -> Mux/3  "<WorldCoordinateX>"
  Bus Selector/3 -> Mux4/3  "<WorldCoordinateY>"
  Bus Selector/4 -> Mux4/4  "<WorldCoordinateY>"
  Bus Selector/1 -> Mux4/1  "<WorldCoordinateY>"
  Bus Selector/2 -> Mux4/2  "<WorldCoordinateY>"
  Mux/1 -> Lane3_X_Part4/1
  Mux4/1 -> Lane3_Y_Part4/1
  Bus Selector6/4 -> Mux5/4  "<WorldCoordinateX>"
  Bus Selector6/3 -> Mux5/3  "<WorldCoordinateX>"
  Bus Selector6/2 -> Mux5/2  "<WorldCoordinateX>"
  Bus Selector6/1 -> Mux5/1  "<WorldCoordinateX>"
  Bus Selector1/3 -> Mux1/3  "<WorldCoordinateY>"
  Bus Selector1/2 -> Mux1/2  "<WorldCoordinateY>"
  Bus Selector1/4 -> Mux1/4  "<WorldCoordinateY>"
  Bus Selector1/1 -> Mux1/1  "<WorldCoordinateY>"
  Mux1/1 -> Lane1_Y_Part4/1
  Mux5/1 -> Lane1_X_Part4/1
  Bus Selector7/2 -> Mux2/2  "<WorldCoordinateX>"
  Bus Selector7/3 -> Mux2/3  "<WorldCoordinateX>"
  Bus Selector7/1 -> Mux2/1  "<WorldCoordinateX>"
  Bus Selector7/4 -> Mux2/4  "<WorldCoordinateX>"
  Bus Selector2/2 -> Mux3/2  "<WorldCoordinateY>"
  Bus Selector2/1 -> Mux3/1  "<WorldCoordinateY>"
  Bus Selector2/3 -> Mux3/3  "<WorldCoordinateY>"
  Bus Selector2/4 -> Mux3/4  "<WorldCoordinateY>"
  Bus Selector3/2 -> Mux6/2  "<WorldCoordinateX>"
  Bus Selector3/1 -> Mux6/1  "<WorldCoordinateX>"
  Bus Selector3/3 -> Mux6/3  "<WorldCoordinateX>"
  Bus Selector3/4 -> Mux6/4  "<WorldCoordinateX>"
  Bus Selector8/1 -> Mux7/1  "<WorldCoordinateY>"
  Bus Selector8/2 -> Mux7/2  "<WorldCoordinateY>"
  Bus Selector8/3 -> Mux7/3  "<WorldCoordinateY>"
  Bus Selector8/4 -> Mux7/4  "<WorldCoordinateY>"
  Mux3/1 -> Lane2_Y_Part4/1
  Mux7/1 -> Lane4_Y_Part4/1
  Mux2/1 -> Lane2_X_Part4/1
  Mux6/1 -> Lane4_X_Part4/1

== system StraightWithLeadingCar_cs/Roewe_550_S_Sedan_1/CarSim_Vehicle/CarSim2PreScan_BUS/Steering/AvoidDivisionByZero ==
  In1 : Inport
  Compare To Zero : simulink/Logic and Bit Operations/Compare To Zero  relop===  OutDataTypeStr=uint8
  Constant : Constant  Value=eps
  Product : Product  RndMeth=Zero
  Sum : Sum
  Out1 : Outport
  wires:
  In1/1 -> Compare To Zero/1, Sum/1
  Sum/1 -> Out1/1
  Product/1 -> Sum/2
  Constant/1 -> Product/2
  Compare To Zero/1 -> Product/1

== system StraightWithLeadingCar_cs/Roewe_550_S_Sedan_1/CarSim_Vehicle/CarSim2PreScan_BUS/Wheel/Convert CarSim to PreScan Wheel Position ==
  SprungMass_Pos_Global[x;y;z][m] : Inport
  SprungMass_Angle_Global[x;y;z][deg] : Inport  Port=2
  CarSim_Pos_FL_Wheel[x;y;z][m] : Inport  Port=3
  CarSim_Pos_FR_Wheel[x;y;z][m] : Inport  Port=4
  CarSim_Pos_RL_Wheel[x;y;z][m] : Inport  Port=5
  CarSim_Pos_RR_Wheel[x;y;z][m] : Inport  Port=6
  Bus Creator1 : BusCreator  Inputs=4
  Demux1 : Demux  Outputs=[3 3 3 3]
  Mux1 : Mux
  Transformation_WheelGlobal2WheelLocal : Subsystem
  PreScanWheel_Pos : Outport
  wires:
  SprungMass_Angle_Global[x;y;z][deg]/1 -> Transformation_WheelGlobal2WheelLocal/2(SprungMass_Angle_Global[x;y;z][deg])
  SprungMass_Pos_Global[x;y;z][m]/1 -> Transformation_WheelGlobal2WheelLocal/1(SprungMass_Pos_Global[x;y;z][m])
  CarSim_Pos_RR_Wheel[x;y;z][m]/1 -> Mux1/4
  CarSim_Pos_RL_Wheel[x;y;z][m]/1 -> Mux1/3
  CarSim_Pos_FR_Wheel[x;y;z][m]/1 -> Mux1/2
  CarSim_Pos_FL_Wheel[x;y;z][m]/1 -> Mux1/1
  Mux1/1 -> Transformation_WheelGlobal2WheelLocal/3(Wheels_Pos_Global[x;y;z][m])
  Bus Creator1/1 -> PreScanWheel_Pos/1  "Linear"
  Demux1/4 -> Bus Creator1/4  "Pos_RR_Wheel_CoorSys_V[x;y;z][m]"
  Demux1/3 -> Bus Creator1/3  "Pos_RL_Wheel_CoorSys_V[x;y;z][m]"
  Demux1/2 -> Bus Creator1/2  "Pos_FR_Wheel_CoorSys_V[x;y;z][m]"
  Demux1/1 -> Bus Creator1/1  "Pos_FL_Wheel_CoorSys_V[x;y;z][m]"
  Transformation_WheelGlobal2WheelLocal/1(Pos_[FL;FR;RL;RR]_Wheel_CoorSys_V[x;y;z][m]) -> Demux1/1

== system StraightWithLeadingCar_cs/Roewe_550_S_Sedan_1/CarSim_Vehicle/CarSim2PreScan_BUS/Wheel/Convert CarSim to PreScan Wheel Rotation ==
  CarSim_Angle_FL_Wheel_CoorSys_V[deg;rev;deg] : Inport
  CarSim_Angle_FR_Wheel_CoorSys_V[deg;rev;deg] : Inport  Port=2
  CarSim_Angle_RL_Wheel_CoorSys_V[deg;rev;deg] : Inport  Port=3
  CarSim_Angle_RR_Wheel_CoorSys_V[deg;rev;deg] : Inport  Port=4
  Angle_Vehicle[x;y;z][deg] : Inport  Port=5
  Bus Creator{,1,3..4} (4 alike) : BusCreator  Inputs=3
  Bus Creator2 : BusCreator  Inputs=4
  Demux{,1..4} (5 alike) : Demux  Outputs=3
  Rev2D{,1..3} (4 alike) : Gain  Gain=360
  Sum{1..4} (4 alike) : Sum  Inputs=+-
  Terminator : Terminator
  Terminator1 : Terminator
  PreScanWheel_Rot : Outport
  wires:
  [VehicleRoll_deg] -> Sum3/2
  Sum3/1 -> Bus Creator4/1  "Angle_Camber_RR_Wheel_CoorSys_V[deg]"
  [VehicleRoll_deg] -> Sum2/2
  Sum1/1 -> Bus Creator1/1  "Angle_Camber_FR_Wheel_CoorSys_V[deg]"
  [VehicleRoll_deg] -> Sum1/2
  [VehicleRoll_deg] -> Sum4/2
  Demux4/3 -> Terminator1/1
  Demux4/2 -> Terminator/1
  Demux4/1 -> [VehicleRoll_deg]
  Angle_Vehicle[x;y;z][deg]/1 -> Demux4/1
  Rev2D3/1 -> Bus Creator4/2  "Angle_Rot_RR_Wheel[deg]"
  Rev2D2/1 -> Bus Creator3/2  "Angle_Rot_RL_Wheel[deg]"
  Rev2D1/1 -> Bus Creator1/2  "Angle_Rot_FR_Wheel[deg]"
  Rev2D/1 -> Bus Creator/2  "Angle_Rot_FL_Wheel[deg]"
  CarSim_Angle_RR_Wheel_CoorSys_V[deg;rev;deg]/1 -> Demux3/1
  CarSim_Angle_RL_Wheel_CoorSys_V[deg;rev;deg]/1 -> Demux2/1
  CarSim_Angle_FR_Wheel_CoorSys_V[deg;rev;deg]/1 -> Demux1/1
  Demux/1 -> Sum4/1  "CarSImAngle_Camber_FL_Wheel_CoorSys_V[deg]"
  Bus Creator2/1 -> PreScanWheel_Rot/1  "Angualr"
  Bus Creator4/1 -> Bus Creator2/4  "Rot_RR_Wheel_CoorSys_V[x;y;z][deg]"
  Bus Creator3/1 -> Bus Creator2/3  "Rot_RL_Wheel_CoorSys_V[x;y;z][deg]"
  Bus Creator1/1 -> Bus Creator2/2  "Rot_FR_Wheel_CoorSys_V[x;y;z][deg]"
  Bus Creator/1 -> Bus Creator2/1  "Rot_FL_Wheel_CoorSys_V[x;y;z][deg]"
  Demux3/3 -> Bus Creator4/3  "Angle_Toe_RR_Wheel_CoorSys_V[deg]"
  Demux1/3 -> Bus Creator1/3  "Angle_Toe_FR_Wheel_CoorSys_V[deg]"
  Demux2/3 -> Bus Creator3/3  "Angle_Toe_RL_Wheel_CoorSys_V[deg]"
  Sum2/1 -> Bus Creator3/1  "Angle_Camber_RL_Wheel_CoorSys_V[deg]"
  Sum4/1 -> Bus Creator/1  "Angle_Camber_FL_Wheel_CoorSys_V[deg]"
  Demux3/2 -> Rev2D3/1  "Angle_Rot_RR_Wheel[rev]"
  Demux3/1 -> Sum3/1  "Angle_Camber_RR_Wheel_CoorSys_V[deg]"
  Demux2/2 -> Rev2D2/1  "Angle_Rot_RL_Wheel[rev]"
  Demux2/1 -> Sum2/1  "Angle_Camber_RL_Wheel_CoorSys_V[deg]"
  Demux1/2 -> Rev2D1/1  "Angle_Rot_FR_Wheel[rev]"
  Demux1/1 -> Sum1/1  "Angle_Camber_FR_Wheel_CoorSys_V[deg]"
  Demux/3 -> Bus Creator/3  "Angle_Toe_FL_Wheel_CoorSys_V[deg]"
  Demux/2 -> Rev2D/1  "Angle_Rot_FL_Wheel[rev]"
  CarSim_Angle_FL_Wheel_CoorSys_V[deg;rev;deg]/1 -> Demux/1

== system StraightWithLeadingCar_cs/Roewe_550_S_Sedan_1/CarSim_Vehicle/TyreContact To Road Information/Contact To Road Information/AvoidDivisionByZero ==
  In1 : Inport
  Compare To Zero : simulink/Logic and Bit Operations/Compare To Zero  relop===  OutDataTypeStr=uint8
  Constant : Constant  Value=eps
  Product : Product  RndMeth=Zero
  Sum : Sum
  Out1 : Outport
  wires:
  In1/1 -> Compare To Zero/1, Sum/1
  Sum/1 -> Out1/1
  Product/1 -> Sum/2
  Constant/1 -> Product/2
  Compare To Zero/1 -> Product/1

== system StraightWithLeadingCar_cs/Roewe_550_S_Sedan_1/CarSim_Vehicle/TyreContact To Road Information/Contact To Road Information/Transformation_PreScan2CarSim ==
  UnitVec_z_CP_CoorSys_PreScan[FL;FR;RL;RR][x;y;z] : Inport
  angles_BODYwrtGLOB_[deg] : Inport  Port=2
  Bus Creator : BusCreator  Inputs=4
  D2R : Gain  Gain=pi/180
  Fcn1 : Fcn  Expr=cos(u(1))*sin(u(2))*sin(u(3))-sin(u(1))*cos(u(3))
  Fcn18 : Fcn  Expr=cos(u(1))*cos(u(2))
  Fcn2 : Fcn  Expr=cos(u(1))*sin(u(2))*cos(u(3))+sin(u(1))*sin(u(3))
  Fcn3 : Fcn  Expr=sin(u(1))*cos(u(2))
  Fcn4 : Fcn  Expr=sin(u(1))*sin(u(2))*sin(u(3))+cos(u(1))*cos(u(3))
  Fcn5 : Fcn  Expr=sin(u(1))*sin(u(2))*cos(u(3))-cos(u(1))*sin(u(3))
  Fcn6 : Fcn  Expr=-sin(u(2))
  Fcn7 : Fcn  Expr=cos(u(2))*sin(u(3))
  Fcn8 : Fcn  Expr=cos(u(2))*cos(u(3))
  Mux2 : Mux  Inputs=9
  Selector : Selector  InputPortWidth=9  IndexOptions=Index vector (dialog)  Indices=[1 2 3]  OutputSizes=1
  Selector1 : Selector  InputPortWidth=9  IndexOptions=Index vector (dialog)  Indices=[4 5 6]  OutputSizes=1
  Selector2 : Selector  InputPortWidth=9  IndexOptions=Index vector (dialog)  Indices=[7 8 9]  OutputSizes=1
  Subsystem : Subsystem
  rot_xyz 2 rot_zyx : Selector  InputPortWidth=3  IndexOptions=Index vector (dialog)  Indices=[3 2 1]  OutputSizes=1
  UnitVec_z_CP_CoorSys _CarSim[FL;FR;RL;RR][x;y;z] : Outport
  wires:
  Fcn18/1 -> Mux2/1
  Fcn3/1 -> Mux2/2
  Fcn6/1 -> Mux2/3
  Fcn1/1 -> Mux2/4
  Fcn4/1 -> Mux2/5
  Fcn7/1 -> Mux2/6
  Fcn2/1 -> Mux2/7
  Fcn5/1 -> Mux2/8
  Fcn8/1 -> Mux2/9
  Mux2/1 -> Selector/1, Selector1/1, Selector2/1  "Inverse RotationMatrix"
  rot_xyz 2 rot_zyx/1 -> Fcn18/1, Fcn3/1, Fcn6/1, Fcn1/1, Fcn4/1, Fcn8/1, Fcn5/1, Fcn2/1, Fcn7/1
  D2R/1 -> rot_xyz 2 rot_zyx/1
  Subsystem/4(UnitVec_z_CP_CoorSys_CarSim[RR][x;y;z]) -> Bus Creator/4
  Subsystem/3(UnitVec_z_CP_CoorSys_CarSim[RL][x;y;z]) -> Bus Creator/3
  Subsystem/2(UnitVec_z_CP_CoorSys_CarSim[FR][x;y;z]) -> Bus Creator/2
  Subsystem/1(UnitVec_z_CP_CoorSys_CarSim[FL][x;y;z]) -> Bus Creator/1
  UnitVec_z_CP_CoorSys_PreScan[FL;FR;RL;RR][x;y;z]/1 -> Subsystem/1(UnitVec_z_CP_CoorSys_PreScan[FL;FR;RL;RR][x;y;z])
  angles_BODYwrtGLOB_[deg]/1 -> D2R/1
  Bus Creator/1 -> UnitVec_z_CP_CoorSys _CarSim[FL;FR;RL;RR][x;y;z]/1
  Selector2/1 -> Subsystem/4(ThirdRow)
  Selector1/1 -> Subsystem/3(SecondRow)
  Selector/1 -> Subsystem/2(FirstRow)

== system StraightWithLeadingCar_cs/Roewe_550_S_Sedan_1/PreScan_RayCast_Contact_Sensor/Vehicle Local to World/state2FullState/Transformation_BODY2GLOBAL1 ==
  POSvector_BODY_[m] : Inport
  angles_BODYwrtGLOB_[rad] : Inport  Port=2
  Dot Product : DotProduct  InputSameDT=on  OutDataTypeStr=Inherit: Inherit via internal rule
  Dot Product1 : DotProduct  InputSameDT=on  OutDataTypeStr=Inherit: Inherit via internal rule
  Dot Product2 : DotProduct  InputSameDT=on  OutDataTypeStr=Inherit: Inherit via internal rule
  Fcn10 : Fcn  Expr=cos(u(1))*sin(u(2))*sin(u(3))-sin(u(1))*cos(u(3))
  Fcn11 : Fcn  Expr=cos(u(1))*sin(u(2))*cos(u(3))+sin(u(1))*sin(u(3))
  Fcn12 : Fcn  Expr=sin(u(1))*cos(u(2))
  Fcn13 : Fcn  Expr=sin(u(1))*sin(u(2))*sin(u(3))+cos(u(1))*cos(u(3))
  Fcn14 : Fcn  Expr=sin(u(1))*sin(u(2))*cos(u(3))-cos(u(1))*sin(u(3))
  Fcn15 : Fcn  Expr=-sin(u(2))
  Fcn16 : Fcn  Expr=cos(u(2))*sin(u(3))
  Fcn17 : Fcn  Expr=cos(u(2))*cos(u(3))
  Fcn9 : Fcn  Expr=cos(u(1))*cos(u(2))
  Mux1 : Mux  Inputs=9
  Mux3 : Mux  Inputs=3
  Selector : Selector  InputPortWidth=9  IndexOptions=Index vector (dialog)  Indices=[1 2 3]  OutputSizes=1
  Selector1 : Selector  InputPortWidth=9  IndexOptions=Index vector (dialog)  Indices=[4 5 6]  OutputSizes=1
  Selector2 : Selector  InputPortWidth=9  IndexOptions=Index vector (dialog)  Indices=[7 8 9]  OutputSizes=1
  rot_xyz 2 rot_zyx : Selector  InputPortWidth=3  IndexOptions=Index vector (dialog)  Indices=[3 2 1]  OutputSizes=1
  POSvector_GLOBAL_[m] : Outport
  wires:
  angles_BODYwrtGLOB_[rad]/1 -> rot_xyz 2 rot_zyx/1
  Mux3/1 -> POSvector_GLOBAL_[m]/1
  rot_xyz 2 rot_zyx/1 -> Fcn17/1, Fcn16/1, Fcn15/1, Fcn14/1, Fcn13/1, Fcn12/1, Fcn11/1, Fcn10/1, Fcn9/1
  Dot Product1/1 -> Mux3/2
  Dot Product2/1 -> Mux3/3
  Selector2/1 -> Dot Product2/2
  Selector1/1 -> Dot Product1/2
  Dot Product/1 -> Mux3/1
  POSvector_BODY_[m]/1 -> Dot Product/1, Dot Product1/1, Dot Product2/1
  Selector/1 -> Dot Product/2
  Mux1/1 -> Selector2/1, Selector1/1, Selector/1  "RotationMatrix"
  Fcn17/1 -> Mux1/9
  Fcn16/1 -> Mux1/8
  Fcn15/1 -> Mux1/7
  Fcn14/1 -> Mux1/6
  Fcn13/1 -> Mux1/5
  Fcn12/1 -> Mux1/4
  Fcn11/1 -> Mux1/3
  Fcn10/1 -> Mux1/2
  Fcn9/1 -> Mux1/1

== system StraightWithLeadingCar_cs/Roewe_550_S_Sedan_1/PreScan_RayCast_Contact_Sensor/Vehicle Local to World/state2FullState/limit roll ==
  RPY : Inport
  Demux : Demux  Outputs=3
  Mux1 : Mux  Inputs=3
  Substitute 90 & 270 deg (and its plurals) : Subsystem
  RPYcor : Outport
  wires:
  Demux/1 -> Substitute 90 & 270 deg (and its plurals)/1(Angle [rad])
  Demux/2 -> Mux1/2
  Demux/3 -> Mux1/3
  RPY/1 -> Demux/1
  Mux1/1 -> RPYcor/1
  Substitute 90 & 270 deg (and its plurals)/1(Subst Angle [rad]) -> Mux1/1

== system StraightWithLeadingCar_cs/Roewe_550_S_Sedan_1/PreScan_RayCast_Contact_Sensor/Wheels Local to World/conv_RotWheelFL/RotMat2AxisAngle ==
  RotMat_Visu : Inport
  Data Type Conversion : DataTypeConversion
  Divide : Product  Inputs=*/
  Gain : Gain  Gain=2
  Mux : Mux  Inputs=3
  Mux1 : Mux  Inputs=2
  Saturation1 : Saturate  UpperLimit=3-0.001  LowerLimit=-1+0.001
  Trigonometric Function : Trigonometry
  U1 : Fcn  Expr=u[6]-u[8]
  U2 : Fcn  Expr=u[7]-u[3]
  U3 : Fcn  Expr=u[2]-u[4]
  U_Phi : Fcn  Expr=u[1]+u[5]+u[9]
  U_Phi1 : Fcn  Expr=acos((u(1)-1)/2)
  U_Phi2 : Fcn  Expr=acos((u(1)-1)/2)
  Angles_Visu : Outport
  wires:
  Data Type Conversion/1 -> Mux1/2
  RotMat_Visu/1 -> U1/1, U2/1, U3/1, U_Phi/1
  Trigonometric Function/1 -> Gain/1
  U1/1 -> Mux/1
  U2/1 -> Mux/2
  U3/1 -> Mux/3
  Mux/1 -> Divide/1
  Gain/1 -> Divide/2
  Mux1/1 -> Angles_Visu/1
  Divide/1 -> Mux1/1
  U_Phi/1 -> U_Phi1/1, Saturation1/1
  U_Phi1/1 -> Data Type Conversion/1
  Saturation1/1 -> U_Phi2/1
  U_Phi2/1 -> Trigonometric Function/1

== system StraightWithLeadingCar_cs/Roewe_550_S_Sedan_1/PreScan_RayCast_Contact_Sensor/Wheels Local to World/conv_RotWheelFR/RotMat2AxisAngle ==
  RotMat_Visu : Inport
  Data Type Conversion : DataTypeConversion
  Divide : Product  Inputs=*/
  Gain : Gain  Gain=2
  Mux : Mux  Inputs=3
  Mux1 : Mux  Inputs=2
  Saturation1 : Saturate  UpperLimit=3-0.001  LowerLimit=-1+0.001
  Trigonometric Function : Trigonometry
  U1 : Fcn  Expr=u[6]-u[8]
  U2 : Fcn  Expr=u[7]-u[3]
  U3 : Fcn  Expr=u[2]-u[4]
  U_Phi : Fcn  Expr=u[1]+u[5]+u[9]
  U_Phi1 : Fcn  Expr=acos((u(1)-1)/2)
  U_Phi2 : Fcn  Expr=acos((u(1)-1)/2)
  Angles_Visu : Outport
  wires:
  U_Phi2/1 -> Trigonometric Function/1
  Saturation1/1 -> U_Phi2/1
  U_Phi1/1 -> Data Type Conversion/1
  U_Phi/1 -> Saturation1/1, U_Phi1/1
  Divide/1 -> Mux1/1
  Mux1/1 -> Angles_Visu/1
  Gain/1 -> Divide/2
  Mux/1 -> Divide/1
  U3/1 -> Mux/3
  U2/1 -> Mux/2
  U1/1 -> Mux/1
  Trigonometric Function/1 -> Gain/1
  RotMat_Visu/1 -> U_Phi/1, U3/1, U2/1, U1/1
  Data Type Conversion/1 -> Mux1/2

== system StraightWithLeadingCar_cs/Roewe_550_S_Sedan_1/PreScan_RayCast_Contact_Sensor/Wheels Local to World/conv_RotWheelRL/RotMat2AxisAngle ==
  RotMat_Visu : Inport
  Data Type Conversion : DataTypeConversion
  Divide : Product  Inputs=*/
  Gain : Gain  Gain=2
  Mux : Mux  Inputs=3
  Mux1 : Mux  Inputs=2
  Saturation1 : Saturate  UpperLimit=3-0.001  LowerLimit=-1+0.001
  Trigonometric Function : Trigonometry
  U1 : Fcn  Expr=u[6]-u[8]
  U2 : Fcn  Expr=u[7]-u[3]
  U3 : Fcn  Expr=u[2]-u[4]
  U_Phi : Fcn  Expr=u[1]+u[5]+u[9]
  U_Phi1 : Fcn  Expr=acos((u(1)-1)/2)
  U_Phi2 : Fcn  Expr=acos((u(1)-1)/2)
  Angles_Visu : Outport
  wires:
  U_Phi2/1 -> Trigonometric Function/1
  Saturation1/1 -> U_Phi2/1
  U_Phi1/1 -> Data Type Conversion/1
  U_Phi/1 -> Saturation1/1, U_Phi1/1
  Divide/1 -> Mux1/1
  Mux1/1 -> Angles_Visu/1
  Gain/1 -> Divide/2
  Mux/1 -> Divide/1
  U3/1 -> Mux/3
  U2/1 -> Mux/2
  U1/1 -> Mux/1
  Trigonometric Function/1 -> Gain/1
  RotMat_Visu/1 -> U_Phi/1, U3/1, U2/1, U1/1
  Data Type Conversion/1 -> Mux1/2

== system StraightWithLeadingCar_cs/Roewe_550_S_Sedan_1/PreScan_RayCast_Contact_Sensor/Wheels Local to World/conv_RotWheelRR/RotMat2AxisAngle ==
  RotMat_Visu : Inport
  Data Type Conversion : DataTypeConversion
  Divide : Product  Inputs=*/
  Gain : Gain  Gain=2
  Mux : Mux  Inputs=3
  Mux1 : Mux  Inputs=2
  Saturation1 : Saturate  UpperLimit=3-0.001  LowerLimit=-1+0.001
  Trigonometric Function : Trigonometry
  U1 : Fcn  Expr=u[6]-u[8]
  U2 : Fcn  Expr=u[7]-u[3]
  U3 : Fcn  Expr=u[2]-u[4]
  U_Phi : Fcn  Expr=u[1]+u[5]+u[9]
  U_Phi1 : Fcn  Expr=acos((u(1)-1)/2)
  U_Phi2 : Fcn  Expr=acos((u(1)-1)/2)
  Angles_Visu : Outport
  wires:
  U_Phi2/1 -> Trigonometric Function/1
  Saturation1/1 -> U_Phi2/1
  U_Phi1/1 -> Data Type Conversion/1
  U_Phi/1 -> Saturation1/1, U_Phi1/1
  Divide/1 -> Mux1/1
  Mux1/1 -> Angles_Visu/1
  Gain/1 -> Divide/2
  Mux/1 -> Divide/1
  U3/1 -> Mux/3
  U2/1 -> Mux/2
  U1/1 -> Mux/1
  Trigonometric Function/1 -> Gain/1
  RotMat_Visu/1 -> U_Phi/1, U3/1, U2/1, U1/1
  Data Type Conversion/1 -> Mux1/2
